simulink model "motionControlModel"  (Simulink 7.7)
settings: Solver=FixedStepDiscrete  SolverMode=SingleTasking  StartTime=0.0  StopTime=60*60*24*365  FixedStep=0.001  RelTol=1e-3
InitFcn:
  | ADB=0;
  | p=1;
  | i1=0;
  | d=0.01;
  | filD=10;
  | 
  | SamT=0.001;
libraries: Diamond16AT_UNAL x1, simulink x1, Stewart_Gough_LibraryV2 x1
settings Model: Creator=LAB_Mecatronica_16  LastModifiedBy=Sebastian  SimulationMode=external  BufferReuse=off
settings DataIOCC: LimitDataPoints=off
settings OptimizationCC: BlockReduction=off  OptimizeBlockIOStorage=off  BufferReuse=off  ExpressionFolding=off  LocalBlockOutputs=off
settings HardwareCC: ProdIntDivRoundTo=Zero  ProdEndianess=LittleEndian  ProdHWDeviceType=Generic->32-bit x86 compatible
settings RTWCC: SystemTargetFile=xpctarget.tlc  TemplateMakefile=xpc_default_tmf  Description=xPC Target  ProcessScript=xpctarget_make_rtw_hook  RTWCompilerOptimization=On
settings xpcTargetCC: TargetFcnLib=ansi_tfl_table_tmw.mat  TargetFunctionLibrary=XPC_BLAS  FunctionExecutionProfile=off  CodeExecutionProfiling=off  ERTCodeCoverageTool=None  ParMdlRefBuildCompliant=on  CombineSignalStateStructs=off  PortableWordSizes=off  xPCTaskExecutionProfile=off  xPCRL32EventNumber=5000  xPCLoadParamSetFile=off  xPCConcurrentTasks=off  xPCEnableSFAnimation=off

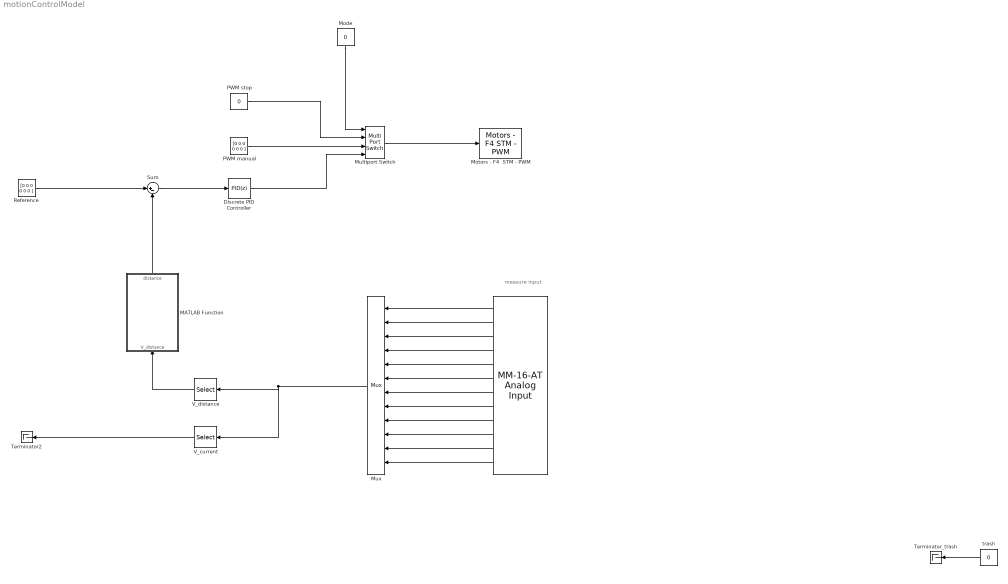
== system motionControlModel ==
  note: measure input
  " " : Diamond16AT_UNAL/Diamond MM-16-AT/MM-16-AT Analog Input  RequirementInfo={} %GIDa_817352d2_1dd7_483d_ad51_97b112d5bcba  configuration=16 Single-ended  firstChan=1  numChans=12  range=0 to 10V  sampleTime=0.001  base=300
  Discrete PID Controller : simulink/Continuous/PID Controller  SystemSampleTime=-1  Controller=PID  TimeDomain=Discrete-time  SampleTime=-1  IntegratorMethod=Forward Euler  FilterMethod=Forward Euler  Form=Parallel  P=1  I=1  D=0  N=100  InitialConditionSource=internal  InitialConditionForIntegrator=0  InitialConditionForFilter=0  ExternalReset=none  LimitOutput=off  UpperSaturationLimit=inf  LowerSaturationLimit=-inf  LinearizeAsGain=off  AntiWindupMode=none  Kb=1  TrackingMode=off  Kt=1  PParamMin=[]  PParamMax=[]  IParamMin=[]  IParamMax=[]  DParamMin=[]  DParamMax=[]  NParamMin=[]  NParamMax=[]  KbParamMin=[]  KbParamMax=[]  KtParamMin=[]  KtParamMax=[]  POutMin=[]  POutMax=[]  IOutMin=[]  IOutMax=[]  DOutMin=[]  DOutMax=[]  NOutMin=[]  NOutMax=[]  KbOutMin=[]  KbOutMax=[]  KtOutMin=[]  KtOutMax=[]  IntegratorOutMin=[]  IntegratorOutMax=[]  FilterOutMin=[]  FilterOutMax=[]  SumOutMin=[]  SumOutMax=[]  SumI1OutMin=[]  SumI1OutMax=[]  SumI2OutMin=[]  SumI2OutMax=[]  SumI3OutMin=[]  SumI3OutMax=[]  SumDOutMin=[]  SumDOutMax=[]  SaturationOutMin=[]  SaturationOutMax=[]  IntegratorContinuousStateAttributes=''  IntegratorStateMustResolveToSignalObject=off  IntegratorRTWStateStorageClass=Auto  FilterContinuousStateAttributes=''  FilterStateMustResolveToSignalObject=off  FilterRTWStateStorageClass=Auto
  MATLAB Function : Stateflow chart  TreatAsAtomicUnit=on
  Mode : Constant  Value=0
  Motors - F4  STM - PWM : Stewart_Gough_LibraryV2/SG - Input//Output/Motors - F4  STM - PWM  SystemSampleTime=-1  Satura=80  SamTime=0.001
  Multiport Switch : MultiPortSwitch  DataPortOrder=Zero-based contiguous  DataPortIndices={1,[2,3]}  DiagnosticForDefault=Warning  zeroidx=on
  Mux : Mux  Inputs=12
  PWM manual : Constant  Value=[0 0 0 0 0 0 ]
  PWM stop : Constant  Value=0
  Reference : Constant  Value=[0 0 0 0 0 0 ]
  Sum : Sum  Inputs=|+-
  Terminator2 : Terminator
  Terminator_trash : Terminator
  V_current : Selector  InputPortWidth=12  IndexOptions=Index vector (dialog)  Indices=[2 4 6 8 10 12]  OutputSizes=1
  V_distance : Selector  InputPortWidth=12  IndexOptions=Index vector (dialog)  Indices=[1 3 5 7 9 11]  OutputSizes=1
  trash : Constant  Value=0
  wires:
  " "/1 -> Mux/1
  " "/2 -> Mux/2
  " "/3 -> Mux/3
  " "/4 -> Mux/4
  " "/5 -> Mux/5
  " "/6 -> Mux/6
  " "/7 -> Mux/7
  " "/8 -> Mux/8
  " "/9 -> Mux/9
  " "/10 -> Mux/10
  " "/11 -> Mux/11
  " "/12 -> Mux/12
  trash/1 -> Terminator_trash/1
  Mode/1 -> Multiport Switch/1
  PWM stop/1 -> Multiport Switch/2
  Multiport Switch/1 -> Motors - F4  STM - PWM/1
  Discrete PID Controller/1 -> Multiport Switch/4
  Reference/1 -> Sum/1
  Sum/1 -> Discrete PID Controller/1
  V_distance/1 -> MATLAB Function/1(V_distance)
  V_current/1 -> Terminator2/1
  MATLAB Function/1(distance) -> Sum/2
  Mux/1 -> V_current/1, V_distance/1
  PWM manual/1 -> Multiport Switch/3

== matlab function MATLAB Function ==
  data: V_distance input double; distance output double
function  distance= input_conversion(V_distance)
%#codegen

distance=V_distance;
